simulink model "Block_SAU"  (R2022a)
settings: Solver=ode23tb  StartTime=0.0  StopTime=10.0  MaxStep=1e-4  RelTol=1e-5
undefined symbols (not defined in the file): DiscIntNeverNeededParam, DT, FI, PI_reg, SAU, ZU
libraries: simulink x2, dspsigattribs x1, dspstat3 x1, dspswit3 x1
settings Model: Creator=админ  LastModifiedBy=админ

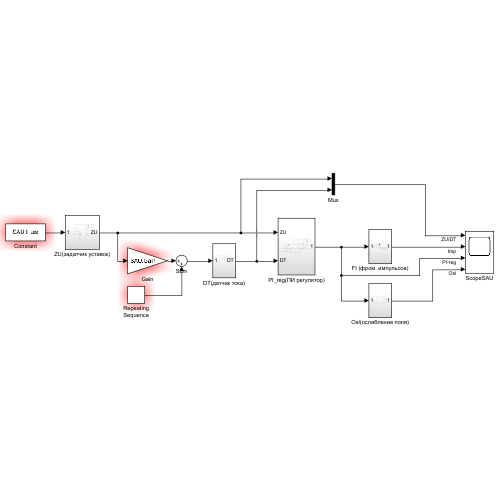
[thumbnail: Simulink's stored preview of the top-level diagram]
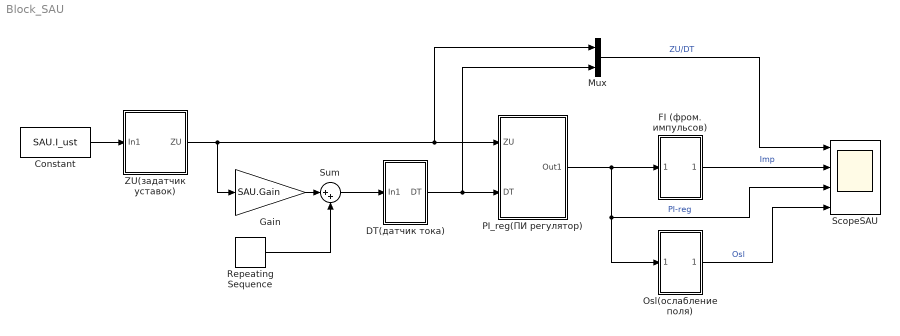
== system Block_SAU ==
  Constant : Constant  Value=SAU.I_ust
  DT(датчик тока) : Subsystem
  FI (фром. импульсов) : Subsystem
  Gain : Gain  Gain=SAU.Gain
  Mux : Mux  Inputs=2
  Osl(ослабление поля) : Subsystem
  PI_reg(ПИ регулятор) : Subsystem
  Repeating Sequence : simulink/Sources/Repeating Sequence  rep_seq_t=SAU.RepSec.Time  rep_seq_y=SAU.RepSec.Output
  ScopeSAU : Scope  NumInputPorts=4
  Sum : Sum  Inputs=|++
  ZU(задатчик уставок) : Subsystem
  wires:
  PI_reg(ПИ регулятор)/1(Out1) -> ScopeSAU/3, Osl(ослабление поля)/1(In1), FI (фром. импульсов)/1(In1)  "PI-reg"
  DT(датчик тока)/1(DT) -> Mux/2, PI_reg(ПИ регулятор)/2(DT)
  ZU(задатчик уставок)/1(ZU) -> Mux/1, PI_reg(ПИ регулятор)/1(ZU), Gain/1
  Constant/1 -> ZU(задатчик уставок)/1(In1)
  Gain/1 -> Sum/1
  Repeating Sequence/1 -> Sum/2
  Sum/1 -> DT(датчик тока)/1(In1)
  Mux/1 -> ScopeSAU/1  "ZU/DT"
  FI (фром. импульсов)/1(Out1) -> ScopeSAU/2  "Imp"
  Osl(ослабление поля)/1(Out1) -> ScopeSAU/4  "Osl"

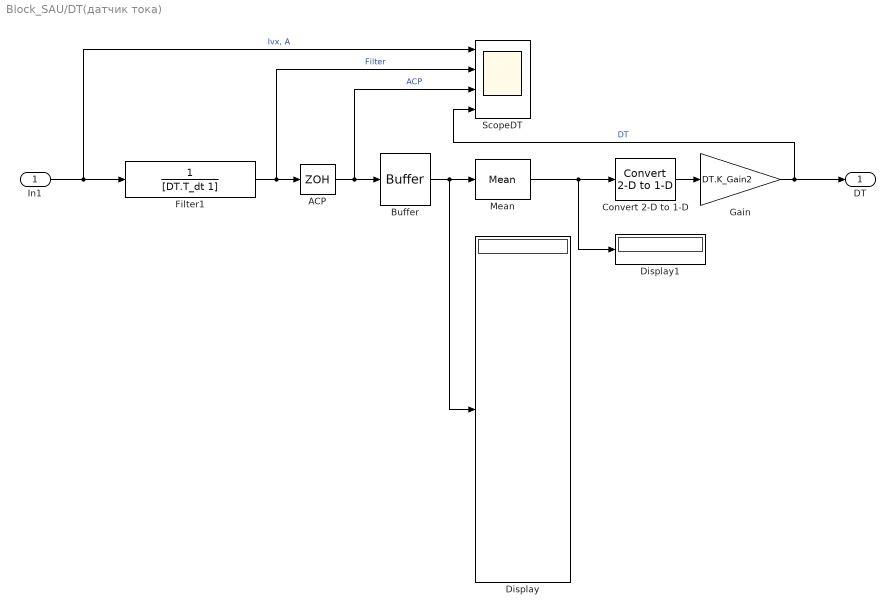
== system Block_SAU/DT(датчик тока) ==
  In1 : Inport
  Buffer : Buffer  N=DT.Buffer_size  OutputFrames=off
  Convert 2-D to 1-D : dspsigattribs/Convert 2-D to 1-D
      settings: SourceProductBaseCode=DS
  Display : Display
  Display1 : Display
  Filter1 : TransferFcn  Denominator=[DT.T_dt 1]
  Gain : Gain  Gain=DT.K_Gain2
  Mean : dspstat3/Mean  run=off  InputProcessing=Columns as channels (frame based)  reset_popup=None  directionMode=Each column  dimension=1  roiEnable=off  roiType=Rectangles  roiPortion=Entire ROI  roiOutput=Individual statistics for each ROI  roiFlag=off  roundingMode=Floor  overflowMode=off  outputDataTypeStr=Inherit: Same as accumulator  outputMin=[]  outputMax=[]  outputLastDataTypeStr=Inherit: Same as accumulator
  ScopeDT : Scope  NumInputPorts=4
  АСР : ZeroOrderHold  SampleTime=DT.T_kv1
  DT : Outport
  wires:
  Filter1/1 -> ScopeDT/2, АСР/1  "Filter"
  АСР/1 -> ScopeDT/3, Buffer/1  "АСР"
  Buffer/1 -> Display/1, Mean/1
  Gain/1 -> DT/1, ScopeDT/4  "DT"
  Mean/1 -> Convert 2-D to 1-D/1, Display1/1
  In1/1 -> Filter1/1, ScopeDT/1  "Ivx, А"
  Convert 2-D to 1-D/1 -> Gain/1

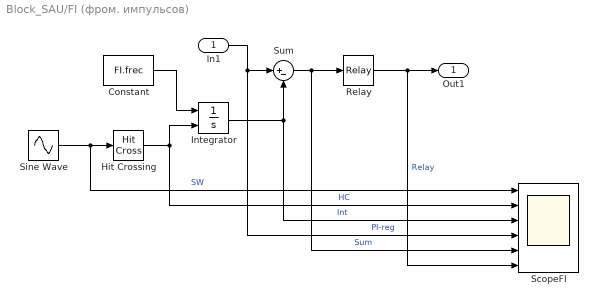
== system Block_SAU/FI (фром. импульсов) ==
  In1 : Inport
  Constant : Constant  Value=FI.frec
  Hit Crossing : HitCross
  Integrator : Integrator  ExternalReset=rising
  Relay : Relay
  ScopeFI : Scope  NumInputPorts=6
  Sine Wave : Sin  Frequency=FI.Sine_Wave.freq  SampleTime=0
  Sum : Sum  Inputs=|+-
  Out1 : Outport
  wires:
  Sine Wave/1 -> ScopeFI/1, Hit Crossing/1  "SW"
  Relay/1 -> Out1/1, ScopeFI/6  "Relay"
  In1/1 -> ScopeFI/4, Sum/1  "PI-reg"
  Hit Crossing/1 -> ScopeFI/2, Integrator/2  "HC"
  Integrator/1 -> ScopeFI/3, Sum/2  "Int"
  Constant/1 -> Integrator/1
  Sum/1 -> ScopeFI/5, Relay/1  "Sum"

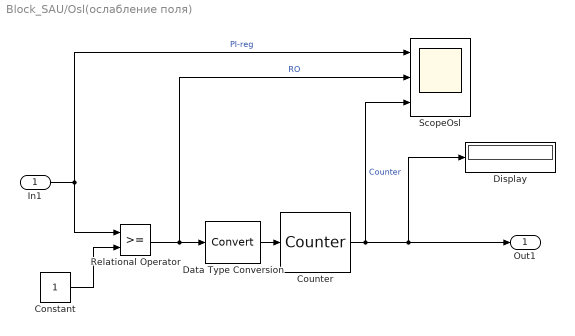
== system Block_SAU/Osl(ослабление поля) ==
  In1 : Inport
  Constant : Constant
  Counter : dspswit3/Counter  Direction=Up  CountEvent=Rising edge  CounterSize=User defined  MaxCount=Osl.Counter_MaxCount  InitialCount=0  Output=Count  HitValue=32  ResetInput=off  SamplesPerFrame=1  Ts=1  CntDtype=double  HitDtype=Logical
  Data Type Conversion : DataTypeConversion  SaturateOnIntegerOverflow=off  RndMeth=Floor
  Display : Display
  Relational Operator : RelationalOperator  OutDataTypeStr=boolean  RndMeth=Simplest  InputSameDT=off
  ScopeOsl : Scope  NumInputPorts=3
  Out1 : Outport
  wires:
  Counter/1 -> Out1/1, Display/1, ScopeOsl/3  "Counter"
  Relational Operator/1 -> ScopeOsl/2, Data Type Conversion/1  "RO"
  Constant/1 -> Relational Operator/2
  In1/1 -> Relational Operator/1, ScopeOsl/1  "PI-reg"
  Data Type Conversion/1 -> Counter/1

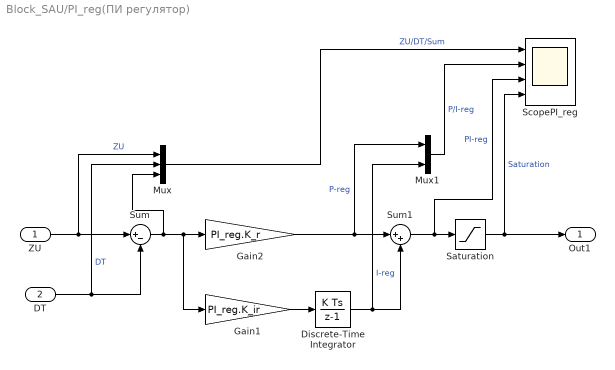
== system Block_SAU/PI_reg(ПИ регулятор) ==
  ZU : Inport
  DT : Inport  Port=2
  Discrete-Time Integrator : DiscreteIntegrator  SampleTime=PI_reg.DTI_st  ICPrevOutput=DiscIntNeverNeededParam  ICPrevScaledInput=DiscIntNeverNeededParam
  Gain1 : Gain  Gain=PI_reg.K_ir
  Gain2 : Gain  Gain=PI_reg.K_r
  Mux : Mux  Inputs=3
  Mux1 : Mux  Inputs=2
  Saturation : Saturate  UpperLimit=PI_reg.StUp_limit  LowerLimit=PI_reg.StLow_limit
  ScopePI_reg : Scope  NumInputPorts=4
  Sum : Sum  Inputs=|+-
  Sum1 : Sum  Inputs=|++
  Out1 : Outport
  wires:
  Sum/1 -> Mux/3, Gain1/1, Gain2/1
  Discrete-Time Integrator/1 -> Mux1/2, Sum1/2  "I-reg"
  Gain2/1 -> Mux1/1, Sum1/1  "P-reg"
  ZU/1 -> Mux/1, Sum/1  "ZU"
  Gain1/1 -> Discrete-Time Integrator/1
  Saturation/1 -> Out1/1, ScopePI_reg/4  "Saturation"
  Sum1/1 -> ScopePI_reg/3, Saturation/1  "PI-reg"
  DT/1 -> Mux/2, Sum/2  "DT"
  Mux/1 -> ScopePI_reg/1  "ZU/DT/Sum"
  Mux1/1 -> ScopePI_reg/2  "P/I-reg"

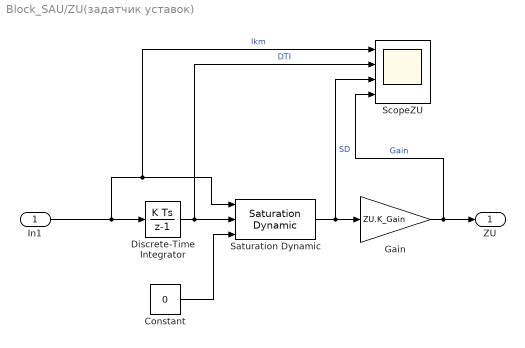
== system Block_SAU/ZU(задатчик уставок) ==
  In1 : Inport
  Constant : Constant  Value=0
  Discrete-Time Integrator : DiscreteIntegrator  gainval=0.5  SampleTime=1/100  ICPrevOutput=DiscIntNeverNeededParam  ICPrevScaledInput=DiscIntNeverNeededParam
  Gain : Gain  Gain=ZU.K_Gain
  Saturation Dynamic : simulink/Discontinuities/Saturation Dynamic  OutMin=[]  OutMax=[]  OutDataTypeStr=Inherit: Same as second input  OutDataType=fixdt(1, 16)  OutScaling=2^-10  DoSatur=off
  ScopeZU : Scope  NumInputPorts=4
  ZU : Outport
  wires:
  Saturation Dynamic/1 -> ScopeZU/3, Gain/1  "SD"
  Discrete-Time Integrator/1 -> ScopeZU/2, Saturation Dynamic/2  "DTI"
  In1/1 -> ScopeZU/1, Saturation Dynamic/1, Discrete-Time Integrator/1  "Ikm"
  Constant/1 -> Saturation Dynamic/3
  Gain/1 -> ScopeZU/4, ZU/1  "Gain"
